simulink model "Kalman"  (R2020a)
settings: Solver=VariableStepAuto  StartTime=0.0  StopTime=117  FixedStep=0.001  RelTol=1e-3
PostLoadFcn:
  | , if any(exist('dsrtsu_mdlpostloadfcn', 'file') == [2, 3, 6]), try dsrtsu_mdlpostloadfcn('Execute', bdroot); catch fprintf('Error in PostLoadFcn (dsrtsu_mdlpostloadfcn) for model "%s":\n %s\n', bdroot, lasterr); end, end,
InitFcn:
  | , if any(exist('rtifpga_mdlclblib', 'file') ~= 0), rtifpga_mdlclblib('Init', bdroot); end,
Description:
  | Standard RTI1401 template.
  | Supported MATLAB version:  R2020a.
settings Model: Tag=RTI1401  DSRTSU_INTERNAL_RTI_VER=580  DSRTSU_INTERNAL_RTI_TYPE=rti1401  RTICANMMDATA=struct('GeneralSetupData',struct('modelroot','C:\Users\soso7\Desktop','generalsettings',struct('filesettings',struct('destfolder',struct('Name','RTICANMM_FILES','Check',1),'buildfolder',struct('Name','.','Check',1),'AbsDestfolder',struct('Name','C:\Users\soso7\Desktop\RTICANMM_FILES'),'AbsBuildfolder',struct('Name','C:\Users\soso7\Desktop'))),'options',struct('addpaths',1,'rmpaths',1,'addtrcexclusion',true,'cannavigator',struct('checkmonitoring',0),'show_usrtrc',0,'use_usrtrc',0),'advanced',struct('options',ones(1,100)),'MPSetup',{{}},'RTI',struct('Type','RTI1401','Ver','7.16','Date','02-May-2021'),'modelname','Kalman','block','Kalman'))  DSRTSU_INTERNAL_RTIFPGA=170  Creator=soso7  LastModifiedBy=soso7
settings DataIOCC: ReturnWorkspaceOutputs=off
settings OptimizationCC: BlockReduction=off  OptimizeBlockIOStorage=off  BufferReuse=off  GlobalBufferReuse=off  ExpressionFolding=off  LocalBlockOutputs=off  OptimizeDataStoreBuffers=off  BusAssignmentInplaceUpdate=off
settings DebuggingCC: PregeneratedLibrarySubsystemCodeDiagnostic=none  ArithmeticOperatorsInVariantConditions=warning
settings HardwareCC: ProdBitPerPointer=32  ProdBitPerSizeT=32  ProdBitPerPtrDiffT=32  ProdLargestAtomicInteger=Integer  ProdEndianess=BigEndian  ProdWordSize=32  ProdLongLongMode=on  ProdHWDeviceType=Custom Processor->Custom  TargetIntDivRoundTo=Zero  TargetEndianess=BigEndian  TargetHWDeviceType=Custom Processor->Custom
settings ModelReferenceCC: EnableParallelModelReferenceBuilds=on  ParallelModelReferenceMATLABWorkerInit=Load Top Model
settings SFSimCC: SimUseLocalCustomCode=off  MATLABDynamicMemAlloc=off  CustomCodeUndefinedFunction=UseInterfaceOnly
settings RTWCC: Description=dSPACE DS1401 Hardware Platform  SystemTargetFile=rti1401.tlc  MakeCommand=make_rti  TemplateMakefile=rti1401.tmf  RTWUseLocalCustomCode=off
settings CodeAppCC: StateflowObjectComments=on
settings STFCustomTargetCC: ParMdlRefBuildCompliant=on  SystemTargetFile=rti1401.tlc
settings GRTTargetCC: TargetLangStandard=C89/C90 (ANSI)  CompOptLevelCompliant=off  ConcurrentExecutionCompliant=off  CombineOutputUpdateFcns=off  MatFileLogging=off  CPPClassGenCompliant=off  UseToolchainInfoCompliant=off
settings ConfigComp: CovMetricSettings=dswe

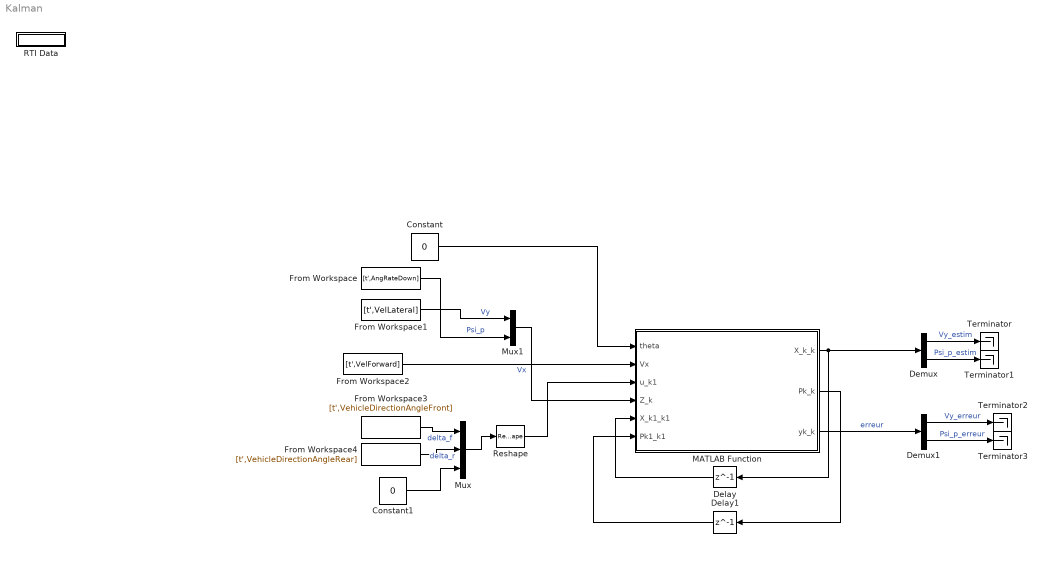
== system Kalman ==
  Constant : Constant  Value=0
  Constant1 : Constant  Value=0
  Delay : Delay  DelayLength=1  InitialCondition=[0 ; 0]
  Delay1 : Delay  DelayLength=1  InitialCondition=eye(2)
  Demux : Demux  Outputs=2
  Demux1 : Demux  Outputs=2
  From Workspace : FromWorkspace  VariableName=[t',AngRateDown]
  From Workspace1 : FromWorkspace  VariableName=[t',VelLateral]
  From Workspace2 : FromWorkspace  VariableName=[t',VelForward]
  From Workspace3 : FromWorkspace  VariableName=[t',VehicleDirectionAngleFront]
  From Workspace4 : FromWorkspace  VariableName=[t',VehicleDirectionAngleRear]
  MATLAB Function : MATLAB Function  TreatAsAtomicUnit=on  SystemSampleTime=0.01
  Mux : Mux  Inputs=3
  Mux1 : Mux  Inputs=2
  RTI Data : Subsystem  Tag=struct('RTIDataServer',struct('RTIDataServerVs','2','RTIModelDescription','struct(''main'',''Kalman'',''sub'',''Kalman'',''isMp'',0)'))  LoadFcn="if exist('rtidc'), try,  rtidc('DataHostBlockClbLoad', gcbh); catch, disp(['Warning: ''LoadFcn'' for RTI Data block failed: ' lasterr]); end, end,"  mask(RTI_DATA_HOST){}
      mask help:
      | RTI Data Block.
      | This block is used by RTI to store internal model-dependent data.
      | Please keep this block on the root level of the model. Deleting this block will result in data loss.
      |
      | NEVER DELETE OR COPY THIS BLOCK!
      settings: CopyFcn="if exist('rtidc'), try,  rtidc('DataHostBlockClbCopy', gcbh); catch, disp(['Warning: ''CopyFcn'' for RTI Data block failed: ' lasterr]); end, end,"  DeleteFcn="if exist('rtidc'), try,  rtidc('DataHostBlockClbDelete', gcbh); catch, disp(['Warning: ''DeleteFcn'' for RTI Data block failed: ' lasterr]); end, end,"  ModelCloseFcn="if exist('rtidc'), try,  rtidc('DataHostBlockClbModelClose', gcbh); catch, disp(['Warning: ''ModelCloseFcn'' for RTI Data block failed: ' lasterr]); end, end,"  PreSaveFcn="if exist('rtidc'), try,  rtidc('DataHostBlockClbPreSave', gcbh); catch, disp(['Warning: ''PreSaveFcn'' for RTI Data block failed: ' lasterr]); end, end,"  PostSaveFcn="if exist('rtidc'), try,  rtidc('DataHostBlockClbPostSave', gcbh); catch, disp(['Warning: ''PostSaveFcn'' for RTI Data block failed: ' lasterr]); end, end,"  NameChangeFcn="if exist('rtidc'), try,  rtidc('DataHostBlockClbNameChange', gcbh); catch, disp(['Warning: ''NameChangeFcn'' for RTI Data block failed: ' lasterr]); end, end,"
      mask Help:
      | RTI Data Block.
      | This block is used by RTI to store internal model-dependent data.
      | Please keep this block on the root level of the model. Deleting this block will result in data loss.
      | 
      | NEVER DELETE OR COPY THIS BLOCK!
      mask Display:
      | text(0.5, 0.5, 'RTI Data', 'HorizontalAlignment', 'center');
      | plot([1 0]);
  Reshape : Reshape  OutputDimensionality=Column vector (2-D)
  Terminator{,1..3} (4 alike) : Terminator
  wires:
  Constant/1 -> MATLAB Function/1(theta)
  From Workspace1/1 -> Mux1/1  "Vy"
  From Workspace2/1 -> MATLAB Function/2(Vx)  "Vx"
  MATLAB Function/2(Pk_k) -> Delay1/1
  MATLAB Function/3(yk_k) -> Demux1/1  "erreur"
  From Workspace3/1 -> Mux/1  "delta_f"
  From Workspace4/1 -> Mux/2  "delta_r"
  Mux/1 -> Reshape/1
  Delay1/1 -> MATLAB Function/6(Pk1_k1)
  Reshape/1 -> MATLAB Function/3(u_k1)
  Constant1/1 -> Mux/3
  Delay/1 -> MATLAB Function/5(X_k1_k1)
  Demux/1 -> Terminator/1  "Vy_estim"
  Demux/2 -> Terminator1/1  "Psi_p_estim"
  MATLAB Function/1(X_k_k) -> Delay/1, Demux/1
  Mux1/1 -> MATLAB Function/4(Z_k)
  From Workspace/1 -> Mux1/2  "Psi_p"
  Demux1/1 -> Terminator2/1  "Vy_erreur"
  Demux1/2 -> Terminator3/1  "Psi_p_erreur"

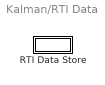
== system Kalman/RTI Data ==
  RTI Data Store : Subsystem  Tag=struct('private',struct('version',struct('dsVer',uint32(2),'dsVerCreation',uint32(2),'RTI',struct('ver','7.16','type','RTI1401')),'access',struct('type','Model','isPerm',1,'created',['12-Jul-2022 18:43:43'],'modified',['25-Jul-2022 11:26:30'],'location','')),'public',struct('main',struct('data',[]),'sub',struct('name','','data',[])))  mask(RTI_DATA_STORE){}
      mask help:
      | RTI Data Store Block. This block is used by RTI to store internal model dependent data. Deleting this block will result in data loss.
      |
      | NEVER DELETE, COPY, OR MODIFY THIS BLOCK!
      mask Help:
      | RTI Data Store Block. This block is used by RTI to store internal model dependent data. Deleting this block will result in data loss.
      | 
      | NEVER DELETE, COPY, OR MODIFY THIS BLOCK!
      mask Display: text(0.5, 0.5, ' ', 'HorizontalAlignment', 'center');

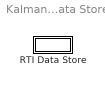
== system Kalman/RTI Data/RTI Data Store ==
  RTI Data Store : Subsystem  mask(RTI_DATA_STORE){}
      mask help:
      | RTI Data Store Block. This block is used by RTI to store internal model dependent data. Deleting this block will result in data loss.
      |
      | NEVER DELETE, COPY, OR MODIFY THIS BLOCK!
      mask Help:
      | RTI Data Store Block. This block is used by RTI to store internal model dependent data. Deleting this block will result in data loss.
      | 
      | NEVER DELETE, COPY, OR MODIFY THIS BLOCK!
      mask Display: text(0.5, 0.5, ' ', 'HorizontalAlignment', 'center');

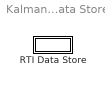
== system Kalman/RTI Data/RTI Data Store/RTI Data Store ==
  RTI Data Store : Subsystem  mask(RTI_DATA_STORE){}
      mask help:
      | RTI Data Store Block. This block is used by RTI to store internal model dependent data. Deleting this block will result in data loss.
      |
      | NEVER DELETE, COPY, OR MODIFY THIS BLOCK!
      mask Help:
      | RTI Data Store Block. This block is used by RTI to store internal model dependent data. Deleting this block will result in data loss.
      | 
      | NEVER DELETE, COPY, OR MODIFY THIS BLOCK!
      mask Display: text(0.5, 0.5, ' ', 'HorizontalAlignment', 'center');

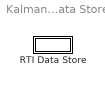
== system Kalman/RTI Data/RTI Data Store/RTI Data Store/RTI Data Store ==
  RTI Data Store : Subsystem  mask(RTI_DATA_STORE){}
      mask help:
      | RTI Data Store Block. This block is used by RTI to store internal model dependent data. Deleting this block will result in data loss.
      |
      | NEVER DELETE, COPY, OR MODIFY THIS BLOCK!
      mask Help:
      | RTI Data Store Block. This block is used by RTI to store internal model dependent data. Deleting this block will result in data loss.
      | 
      | NEVER DELETE, COPY, OR MODIFY THIS BLOCK!
      mask Display: text(0.5, 0.5, ' ', 'HorizontalAlignment', 'center');

== system Kalman/RTI Data/RTI Data Store/RTI Data Store/RTI Data Store/RTI Data Store ==

== matlab function Kalman/MATLAB Function ==
  data: X_k_k output; Pk_k output; theta input; Vx input; u_k1 input; Z_k input; yk_k output; X_k1_k1 input; Pk1_k1 input
function [X_k_k,Pk_k,yk_k]  = fcn(theta,Vx,u_k1,Z_k,X_k1_k1,Pk1_k1)
persistent init;



%% Definition des variables
C_alpha_f = 5.30*10^4; %4.3 * 10^5;  %97035; % Cornering stiffnesses
C_alpha_r = 5.30*10^4; %4.3 * 10^5; %-1.6505e+01; %91631;
C_sig_f = 2.12E+03; %1.4721e+01; %3*10^3;  % Longitudinal stiffnesses
C_sig_r = 2.12E+03; %1.4721e+01; %3*10^3;


Lf = 1.135;
Lr = 1.115;
Lw = 1.330;

R_eff = 0.375;

Iz = 746077895.82505 *10^(-3*2); %3503; %m*Lf^2;
Iw = 1985555 * 10^(-6); %983698 *10-6; %400;

m = 2000; %masse

%% Variables nn constantes dans A
if ((Vx <= 0.1) && (Vx >=0))
   Vx_1 = 0.1;
elseif ((Vx >= -0.1) && (Vx <0))
    Vx_1 = -0.1;
else
   Vx_1 = Vx;
end
% Vx_1= sign(Vx)* max(abs(Vx),0.1);
% u_1 = [Psi_p ; Vy];


%% Definition matrice A
A_y =[-(2*C_alpha_f+2*C_alpha_r)/(m*Vx_1)    -Vx-(2*C_alpha_f*Lf-2*C_alpha_r*Lr)/(m*Vx_1)];
A_psi =[-(2*C_alpha_f*Lf-2*C_alpha_r*Lr)/(Iz*Vx_1)    -(2*C_alpha_f*Lf^2+2*C_alpha_r*Lr^2)/(Iz*Vx_1)];


A = [A_y ; A_psi];
%% Definition matrice B
B =[ (2*C_alpha_f)/m          (2*C_alpha_r)/m              0;
           (2*C_alpha_f*Lf)/Iz      -(2*C_alpha_r*Lr)/Iz         1/Iz];

%% Calcul de P
% g = 9.81; 
% P = -theta*g;

%% Definition de C
C =[1 0 ; 0 1];
D = zeros(2,3);

% Changement de nom
A_k1 = A;
B_k1 = B;
C_k1 = C;
D_k1 = D;


%%%%%%%%%%%%%% Kalman %%%%%%%%%%%%%%%%%%%%%%%%%%%%%%%%%%%%%%%%%%%%%
%% Init

% if isempty(init)
% %     X_k1_k1 = [0 ; 0];
%     Pk1_k1 = eye(2); %cov(X_k1_k1,X_k1_k1); 
%     
%     init = 1;
% end


%% need definir le bruit

% v = wgn(1,200,1E-5,1,23341,'linear');
% n =wgn(1,200,1E-7,1,23341,'linear');

% c = 1.0019e-05;
c1 = 1.0000e-04;
c2 = 8.3729e-06; % Supposes constants
d = c1*10^(-2);
R_nk1 = [c1 0 ; 0 c2]; %cov(v); % coVariance du bruit de mesure
R_vk1 = [d 0 ; 0 d]; %cov(n); % coVariance du bruit de process



% Prediction
X_k_k1 = A_k1 * X_k1_k1 + B_k1 * u_k1;
Pk_k1 = A_k1 * Pk1_k1 * A_k1' + R_vk1; % Rvk : Q

%Correction
y_k = Z_k - C_k1*X_k_k1;

S_k = C_k1*Pk_k1*C_k1' + R_nk1; % R_nk : R
K_k = Pk_k1*C_k1'*S_k^(-1);
X_k_k = X_k_k1 + K_k*y_k; % Z c'est y=Cx + Du, y c'est l'erreur
Pk_k = (eye(2) - K_k*C_k1)*Pk_k1; %I de quelle taille?

yk_k = Z_k - C_k1*X_k_k;
